simulink library "Tetris_Lib"  (R2023a)
settings: Solver=ode45  StartTime=0.0  StopTime=10.0  RelTol=1e-3  EnableMultiTasking=on
libraries: simulink_extras x33, $bdroot x16, Bit_Multiplexers_Lib x9, Decoders_Lib x4
(part 1 of 2)
settings Model: Creator=Jozko Mrkvicka  LastModifiedBy=Jozko Mrkvicka
settings SolverCC: AlgebraicLoopSolver=TrustRegion
settings DataIOCC: LimitDataPoints=on  ReturnWorkspaceOutputs=off
settings OptimizationCC: LifeSpan=inf
settings DebuggingCC: UnconnectedInputMsg=warning  UnconnectedOutputMsg=warning  UnconnectedLineMsg=warning  AllowSymbolicDim=off  SFUnexpectedBacktrackingDiag=warning  SFNoUnconditionalDefaultTransitionDiag=warning  ArithmeticOperatorsInVariantConditions=warning
settings ModelReferenceCC: EnableRefExpFcnMdlSchedulingChecks=on
settings SFSimCC: SimUseLocalCustomCode=off  CustomCodeUndefinedFunction=UseInterfaceOnly
settings RTWCC: RTWUseLocalCustomCode=off
settings CodeAppCC: StateflowObjectComments=on
settings GRTTargetCC: TargetLangStandard=C89/C90 (ANSI)
settings ConfigComp: CovMetricSettings=dw  CovSaveCumulativeToWorkspaceVar=on  CovSaveSingleToWorkspaceVar=on  CovExternalEMLEnable=off

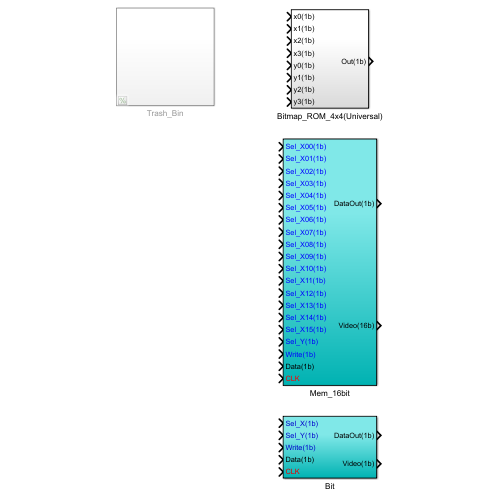
[thumbnail: Simulink's stored preview of the top-level diagram]
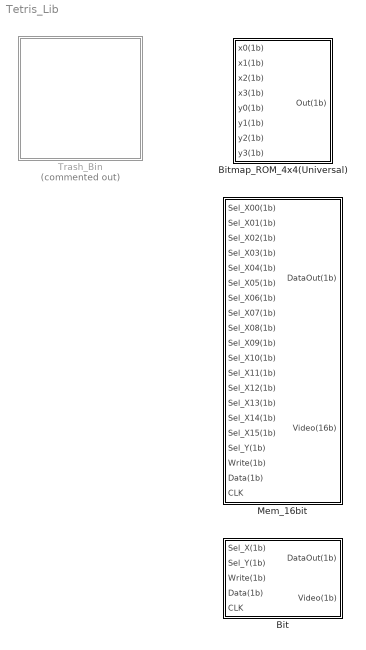
== system Tetris_Lib ==
  Bit : Subsystem
  Bitmap_ROM_4x4(Universal) : Subsystem
  Mem_16bit : Subsystem
  Trash_Bin : Subsystem  Commented=on

== system Tetris_Lib/Bit ==
  Sel_X(1b) : Inport  OutDataTypeStr=boolean
  Sel_Y(1b) : Inport  Port=2  OutDataTypeStr=boolean
  Write(1b) : Inport  Port=3  OutDataTypeStr=boolean
  Data(1b) : Inport  Port=4  OutDataTypeStr=boolean
  CLK : Inport  Port=5  OutDataTypeStr=double
  J-K Flip-Flop : simulink_extras/Flip Flops/J-K Flip-Flop  initial_condition=0
  Logical Operator : Logic  Operator=NOT  IconShape=distinctive  AllPortsSameDT=off  OutDataTypeStr=boolean
  Logical Operator1 : Logic  Inputs=3  IconShape=distinctive  AllPortsSameDT=off  OutDataTypeStr=boolean
  Logical Operator2 : Logic  Inputs=3  IconShape=distinctive  AllPortsSameDT=off  OutDataTypeStr=boolean
  Logical Operator3 : Logic  IconShape=distinctive  AllPortsSameDT=off  OutDataTypeStr=boolean
  Logical Operator4 : Logic  IconShape=distinctive  AllPortsSameDT=off  OutDataTypeStr=boolean
  Terminator : Terminator
  DataOut(1b) : Outport
  Video(1b) : Outport  Port=2
  wires:
  Write(1b)/1 -> Logical Operator1/2, Logical Operator2/2
  Logical Operator3/1 -> Logical Operator1/1, Logical Operator2/1, Logical Operator4/1
  Logical Operator4/1 -> DataOut(1b)/1
  Data(1b)/1 -> Logical Operator/1, Logical Operator1/3
  J-K Flip-Flop/2 -> Terminator/1
  J-K Flip-Flop/1 -> Logical Operator4/2, Video(1b)/1
  CLK/1 -> J-K Flip-Flop/2
  Logical Operator/1 -> Logical Operator2/3
  Logical Operator1/1 -> J-K Flip-Flop/1
  Logical Operator2/1 -> J-K Flip-Flop/3
  Sel_Y(1b)/1 -> Logical Operator3/2
  Sel_X(1b)/1 -> Logical Operator3/1

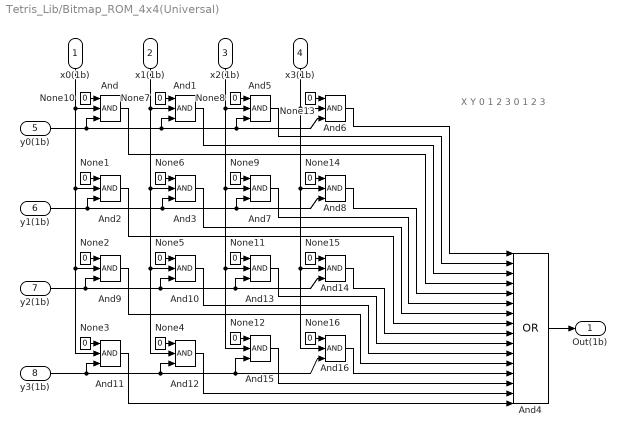
== system Tetris_Lib/Bitmap_ROM_4x4(Universal) ==
  note: X
      |
      | Y
      |
      | 0
      | 1
      | 2
      | 3
      |
      | 0
      |
      | 1
      |
      | 2
      |
      | 3
  x0(1b) : Inport
  x1(1b) : Inport  Port=2
  x2(1b) : Inport  Port=3
  x3(1b) : Inport  Port=4
  y0(1b) : Inport  Port=5
  y1(1b) : Inport  Port=6
  y2(1b) : Inport  Port=7
  y3(1b) : Inport  Port=8
  And{,1..3,5..16} (16 alike) : Logic  Inputs=3  IconShape=distinctive  AllPortsSameDT=off  OutDataTypeStr=boolean
  And4 : Logic  Operator=OR  Inputs=16  IconShape=distinctive  AllPortsSameDT=off  OutDataTypeStr=boolean
  None{1..16} (16 alike) : Constant  Value=0  OutDataTypeStr=boolean
  Out(1b) : Outport
  wires:
  y0(1b)/1 -> And/3, And1/3, And6/3, And5/3
  y1(1b)/1 -> And2/3, And3/3, And8/3, And7/3
  x0(1b)/1 -> And/2, And2/2, And11/2, And9/2
  x1(1b)/1 -> And1/2, And3/2, And12/2, And10/2
  And4/1 -> Out(1b)/1
  x2(1b)/1 -> And5/2, And7/2, And15/2, And13/2
  x3(1b)/1 -> And6/2, And8/2, And16/2, And14/2
  y2(1b)/1 -> And9/3, And10/3, And14/3, And13/3
  y3(1b)/1 -> And11/3, And12/3, And16/3, And15/3
  And6/1 -> And4/1
  And5/1 -> And4/2
  And1/1 -> And4/3
  And/1 -> And4/4
  And8/1 -> And4/5
  And7/1 -> And4/6
  And3/1 -> And4/7
  And2/1 -> And4/8
  And14/1 -> And4/9
  And13/1 -> And4/10
  And10/1 -> And4/11
  And9/1 -> And4/12
  And16/1 -> And4/13
  And15/1 -> And4/14
  And12/1 -> And4/15
  And11/1 -> And4/16
  None10/1 -> And/1
  None1/1 -> And2/1
  None2/1 -> And9/1
  None3/1 -> And11/1
  None4/1 -> And12/1
  None5/1 -> And10/1
  None6/1 -> And3/1
  None7/1 -> And1/1
  None8/1 -> And5/1
  None9/1 -> And7/1
  None11/1 -> And13/1
  None12/1 -> And15/1
  None13/1 -> And6/1
  None14/1 -> And8/1
  None15/1 -> And14/1
  None16/1 -> And16/1

== system Tetris_Lib/Mem_16bit ==
  Sel_X00(1b) : Inport
  Sel_X01(1b) : Inport  Port=2
  Sel_X02(1b) : Inport  Port=3
  Sel_X03(1b) : Inport  Port=4
  Sel_X04(1b) : Inport  Port=5
  Sel_X05(1b) : Inport  Port=6
  Sel_X06(1b) : Inport  Port=7
  Sel_X07(1b) : Inport  Port=8
  Sel_X08(1b) : Inport  Port=9
  Sel_X09(1b) : Inport  Port=10
  Sel_X10(1b) : Inport  Port=11
  Sel_X11(1b) : Inport  Port=12
  Sel_X12(1b) : Inport  Port=13
  Sel_X13(1b) : Inport  Port=14
  Sel_X14(1b) : Inport  Port=15
  Sel_X15(1b) : Inport  Port=16
  Sel_Y(1b) : Inport  Port=17
  Write(1b) : Inport  Port=18
  Data(1b) : Inport  Port=19
  CLK : Inport  Port=20
  Bit{,1..15} (16 alike) : $bdroot/Bit  SystemSampleTime=-1  VariantActivationTime=update diagram  Latency=0  AutoFrameSizeCalculation=off
  Bus Creator3 : BusCreator  Inputs=16
  Logical Operator61 : Logic  Operator=OR  Inputs=16  IconShape=distinctive  AllPortsSameDT=off  OutDataTypeStr=boolean
  DataOut(1b) : Outport
  Video(16b) : Outport  Port=2
  wires:
  Sel_Y(1b)/1 -> Bit/2, Bit15/2, Bit14/2, Bit13/2, Bit12/2, Bit11/2, Bit10/2, Bit9/2, Bit8/2, Bit7/2, Bit6/2, Bit5/2, Bit4/2, Bit3/2, Bit2/2, Bit1/2
  Data(1b)/1 -> Bit/4, Bit10/4, Bit11/4, Bit15/4, Bit14/4, Bit13/4, Bit12/4, Bit9/4, Bit8/4, Bit7/4, Bit6/4, Bit5/4, Bit4/4, Bit3/4, Bit2/4, Bit1/4
  CLK/1 -> Bit/5, Bit15/5, Bit14/5, Bit13/5, Bit12/5, Bit11/5, Bit10/5, Bit9/5, Bit8/5, Bit7/5, Bit6/5, Bit5/5, Bit4/5, Bit3/5, Bit2/5, Bit1/5
  Sel_X00(1b)/1 -> Bit/1
  Sel_X01(1b)/1 -> Bit1/1
  Sel_X02(1b)/1 -> Bit2/1
  Sel_X03(1b)/1 -> Bit3/1
  Sel_X04(1b)/1 -> Bit4/1
  Sel_X05(1b)/1 -> Bit5/1
  Sel_X06(1b)/1 -> Bit6/1
  Sel_X07(1b)/1 -> Bit7/1
  Sel_X08(1b)/1 -> Bit8/1
  Sel_X09(1b)/1 -> Bit9/1
  Sel_X10(1b)/1 -> Bit10/1
  Sel_X11(1b)/1 -> Bit11/1
  Sel_X12(1b)/1 -> Bit12/1
  Sel_X13(1b)/1 -> Bit13/1
  Sel_X14(1b)/1 -> Bit14/1
  Sel_X15(1b)/1 -> Bit15/1
  Write(1b)/1 -> Bit/3, Bit15/3, Bit14/3, Bit13/3, Bit12/3, Bit11/3, Bit10/3, Bit9/3, Bit8/3, Bit7/3, Bit6/3, Bit5/3, Bit4/3, Bit3/3, Bit2/3, Bit1/3
  Bit15/1 -> Logical Operator61/1
  Bit14/1 -> Logical Operator61/2
  Bit13/1 -> Logical Operator61/3
  Bit12/1 -> Logical Operator61/4
  Bit11/1 -> Logical Operator61/5
  Bit10/1 -> Logical Operator61/6
  Bit9/1 -> Logical Operator61/7
  Bit8/1 -> Logical Operator61/8
  Bit7/1 -> Logical Operator61/9
  Bit6/1 -> Logical Operator61/10
  Bit5/1 -> Logical Operator61/11
  Bit4/1 -> Logical Operator61/12
  Bit3/1 -> Logical Operator61/13
  Bit2/1 -> Logical Operator61/15
  Bit1/1 -> Logical Operator61/14
  Bit/1 -> Logical Operator61/16
  Bit15/2 -> Bus Creator3/16
  Bit14/2 -> Bus Creator3/15
  Bit13/2 -> Bus Creator3/14
  Bit12/2 -> Bus Creator3/13
  Bit11/2 -> Bus Creator3/12
  Bit10/2 -> Bus Creator3/11
  Bit9/2 -> Bus Creator3/10
  Bit8/2 -> Bus Creator3/9
  Bit7/2 -> Bus Creator3/8
  Bit6/2 -> Bus Creator3/7
  Bit5/2 -> Bus Creator3/6
  Bit4/2 -> Bus Creator3/5
  Bit3/2 -> Bus Creator3/4
  Bit2/2 -> Bus Creator3/3
  Bit1/2 -> Bus Creator3/2
  Bit/2 -> Bus Creator3/1
  Logical Operator61/1 -> DataOut(1b)/1
  Bus Creator3/1 -> Video(16b)/1

== system Tetris_Lib/Trash_Bin ==
  L1-Shape : Subsystem  Commented=on
  L2-Shape : Subsystem  Commented=on
  NOT_USED_I-Shape : Subsystem  Commented=on
  NOT_USED_O-Shape : Subsystem  Commented=on
  Shape_Bitmaps : Subsystem
  Subsystem1 : Subsystem
  T-Shape : Subsystem  Commented=on
  Z1-Shape : Subsystem  Commented=on
  Z2-Shape : Subsystem  Commented=on

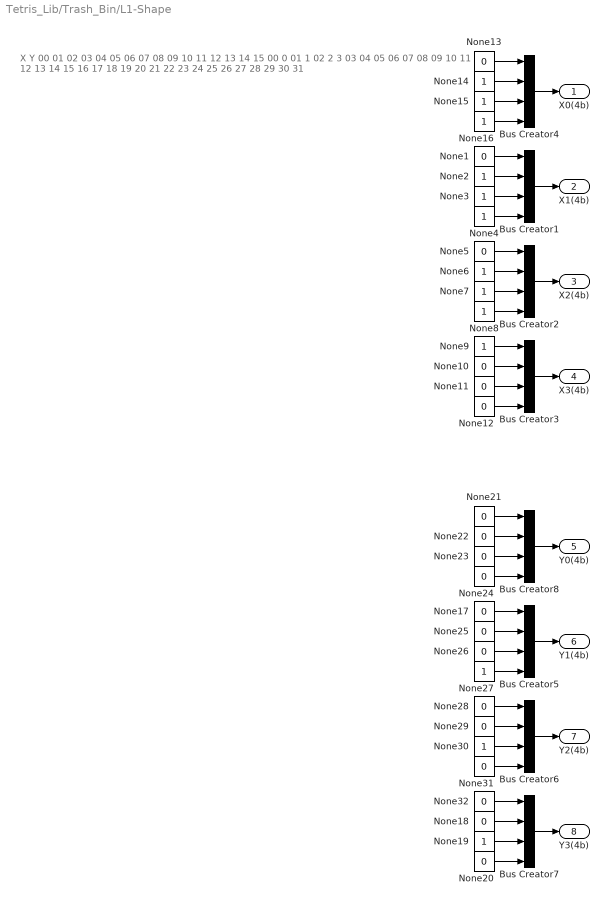
== system Tetris_Lib/Trash_Bin/L1-Shape ==
  note: X
      |
      | Y
      |
      | 00
      | 01
      | 02
      | 03
      | 04
      | 05
      | 06
      | 07
      | 08
      | 09
      | 10
      | 11
      | 12
      | 13
      | 14
      | 15
      |
      | 00
      |
      | 0
      |
      | 01
      |
      | 1
      |
      | 02
      |
      | 2
      | 3
      |
      | 03
      |
      | 04
      |
      | 05
      |
      | 06
      |
      | 07
      |
      | 08
      |
      | 09
      |
      | 10
      |
      | 11
      |
      | 12
      |
      | 13
      |
      | 14
      |
      | 15
      |
      | 16
      |
      | 17
      |
      | 18
      |
      | 19
      |
      | 20
      |
      | 21
      |
      | 22
      |
      | 23
      |
      | 24
      |
      | 25
      |
      | 26
      |
      | 27
      |
      | 28
      |
      | 29
      |
      | 30
      |
      | 31
  Bus Creator{1..8} (8 alike) : BusCreator  Inputs=4
  None{1,5,10..13,17..18,20..26,28..29,31..32} (19 alike) : Constant  Value=0  OutDataTypeStr=boolean
  None{2..4,6..9,14..16,19,27,30} (13 alike) : Constant  OutDataTypeStr=boolean
  X0(4b) : Outport
  X1(4b) : Outport  Port=2
  X2(4b) : Outport  Port=3
  X3(4b) : Outport  Port=4
  Y0(4b) : Outport  Port=5
  Y1(4b) : Outport  Port=6
  Y2(4b) : Outport  Port=7
  Y3(4b) : Outport  Port=8
  wires:
  None24/1 -> Bus Creator8/4
  None23/1 -> Bus Creator8/3
  None22/1 -> Bus Creator8/2
  None21/1 -> Bus Creator8/1
  Bus Creator8/1 -> Y0(4b)/1
  None20/1 -> Bus Creator7/4
  None19/1 -> Bus Creator7/3
  None18/1 -> Bus Creator7/2
  None32/1 -> Bus Creator7/1
  Bus Creator7/1 -> Y3(4b)/1
  None31/1 -> Bus Creator6/4
  None30/1 -> Bus Creator6/3
  None29/1 -> Bus Creator6/2
  None28/1 -> Bus Creator6/1
  Bus Creator6/1 -> Y2(4b)/1
  None27/1 -> Bus Creator5/4
  None26/1 -> Bus Creator5/3
  None25/1 -> Bus Creator5/2
  None17/1 -> Bus Creator5/1
  Bus Creator5/1 -> Y1(4b)/1
  None16/1 -> Bus Creator4/4
  None15/1 -> Bus Creator4/3
  None14/1 -> Bus Creator4/2
  None13/1 -> Bus Creator4/1
  Bus Creator4/1 -> X0(4b)/1
  None12/1 -> Bus Creator3/4
  None11/1 -> Bus Creator3/3
  None10/1 -> Bus Creator3/2
  None9/1 -> Bus Creator3/1
  Bus Creator3/1 -> X3(4b)/1
  None8/1 -> Bus Creator2/4
  None7/1 -> Bus Creator2/3
  None6/1 -> Bus Creator2/2
  None5/1 -> Bus Creator2/1
  Bus Creator2/1 -> X2(4b)/1
  None4/1 -> Bus Creator1/4
  None3/1 -> Bus Creator1/3
  None2/1 -> Bus Creator1/2
  None1/1 -> Bus Creator1/1
  Bus Creator1/1 -> X1(4b)/1

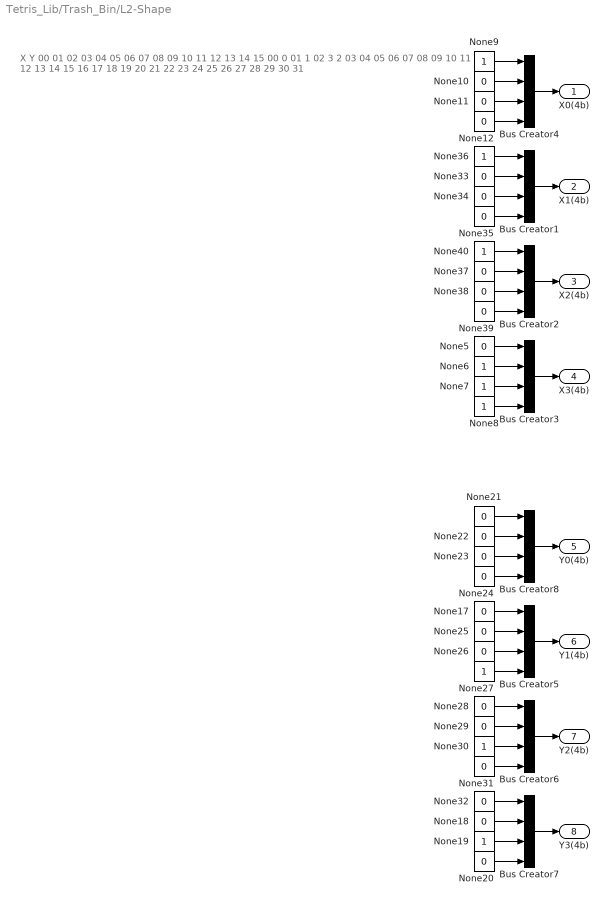
== system Tetris_Lib/Trash_Bin/L2-Shape ==
  note: X
      |
      | Y
      |
      | 00
      | 01
      | 02
      | 03
      | 04
      | 05
      | 06
      | 07
      | 08
      | 09
      | 10
      | 11
      | 12
      | 13
      | 14
      | 15
      |
      | 00
      |
      | 0
      |
      | 01
      |
      | 1
      |
      | 02
      |
      | 3
      | 2
      |
      | 03
      |
      | 04
      |
      | 05
      |
      | 06
      |
      | 07
      |
      | 08
      |
      | 09
      |
      | 10
      |
      | 11
      |
      | 12
      |
      | 13
      |
      | 14
      |
      | 15
      |
      | 16
      |
      | 17
      |
      | 18
      |
      | 19
      |
      | 20
      |
      | 21
      |
      | 22
      |
      | 23
      |
      | 24
      |
      | 25
      |
      | 26
      |
      | 27
      |
      | 28
      |
      | 29
      |
      | 30
      |
      | 31
  Bus Creator{1..8} (8 alike) : BusCreator  Inputs=4
  None{5,10..12,17..18,20..26,28..29,31..35,37..39} (23 alike) : Constant  Value=0  OutDataTypeStr=boolean
  None{6..9,19,27,30,36,40} (9 alike) : Constant  OutDataTypeStr=boolean
  X0(4b) : Outport
  X1(4b) : Outport  Port=2
  X2(4b) : Outport  Port=3
  X3(4b) : Outport  Port=4
  Y0(4b) : Outport  Port=5
  Y1(4b) : Outport  Port=6
  Y2(4b) : Outport  Port=7
  Y3(4b) : Outport  Port=8
  wires:
  None24/1 -> Bus Creator8/4
  None23/1 -> Bus Creator8/3
  None22/1 -> Bus Creator8/2
  None21/1 -> Bus Creator8/1
  Bus Creator8/1 -> Y0(4b)/1
  None20/1 -> Bus Creator7/4
  None19/1 -> Bus Creator7/3
  None18/1 -> Bus Creator7/2
  None32/1 -> Bus Creator7/1
  Bus Creator7/1 -> Y3(4b)/1
  None31/1 -> Bus Creator6/4
  None30/1 -> Bus Creator6/3
  None29/1 -> Bus Creator6/2
  None28/1 -> Bus Creator6/1
  Bus Creator6/1 -> Y2(4b)/1
  None27/1 -> Bus Creator5/4
  None26/1 -> Bus Creator5/3
  None25/1 -> Bus Creator5/2
  None17/1 -> Bus Creator5/1
  Bus Creator5/1 -> Y1(4b)/1
  None12/1 -> Bus Creator4/4
  None11/1 -> Bus Creator4/3
  None10/1 -> Bus Creator4/2
  None9/1 -> Bus Creator4/1
  Bus Creator4/1 -> X0(4b)/1
  None8/1 -> Bus Creator3/4
  None7/1 -> Bus Creator3/3
  None6/1 -> Bus Creator3/2
  None5/1 -> Bus Creator3/1
  Bus Creator3/1 -> X3(4b)/1
  None39/1 -> Bus Creator2/4
  None38/1 -> Bus Creator2/3
  None37/1 -> Bus Creator2/2
  None40/1 -> Bus Creator2/1
  Bus Creator2/1 -> X2(4b)/1
  None35/1 -> Bus Creator1/4
  None34/1 -> Bus Creator1/3
  None33/1 -> Bus Creator1/2
  None36/1 -> Bus Creator1/1
  Bus Creator1/1 -> X1(4b)/1

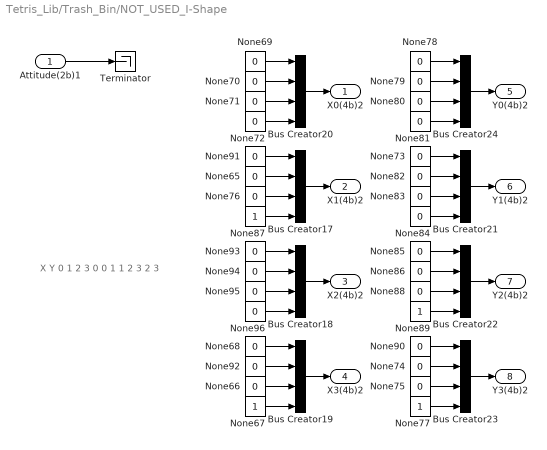
== system Tetris_Lib/Trash_Bin/NOT_USED_I-Shape ==
  note: X
      |
      | Y
      |
      | 0
      | 1
      | 2
      | 3
      |
      | 0
      | 0
      | 1
      |
      | 1
      | 2
      | 3
      |
      | 2
      |
      | 3
  Attitude(2b)1 : Inport
  Bus Creator{17..24} (8 alike) : BusCreator  Inputs=4
  None{65..66,68..76,78..86,88,90..96} (28 alike) : Constant  Value=0  OutDataTypeStr=boolean
  None{67,77,87,89} (4 alike) : Constant  OutDataTypeStr=boolean
  Terminator : Terminator
  X0(4b)2 : Outport
  X1(4b)2 : Outport  Port=2
  X2(4b)2 : Outport  Port=3
  X3(4b)2 : Outport  Port=4
  Y0(4b)2 : Outport  Port=5
  Y1(4b)2 : Outport  Port=6
  Y2(4b)2 : Outport  Port=7
  Y3(4b)2 : Outport  Port=8
  wires:
  Attitude(2b)1/1 -> Terminator/1
  None81/1 -> Bus Creator24/4
  None80/1 -> Bus Creator24/3
  None79/1 -> Bus Creator24/2
  None78/1 -> Bus Creator24/1
  Bus Creator24/1 -> Y0(4b)2/1
  None77/1 -> Bus Creator23/4
  None75/1 -> Bus Creator23/3
  None74/1 -> Bus Creator23/2
  None90/1 -> Bus Creator23/1
  Bus Creator23/1 -> Y3(4b)2/1
  None89/1 -> Bus Creator22/4
  None88/1 -> Bus Creator22/3
  None86/1 -> Bus Creator22/2
  None85/1 -> Bus Creator22/1
  Bus Creator22/1 -> Y2(4b)2/1
  None84/1 -> Bus Creator21/4
  None83/1 -> Bus Creator21/3
  None82/1 -> Bus Creator21/2
  None73/1 -> Bus Creator21/1
  Bus Creator21/1 -> Y1(4b)2/1
  None72/1 -> Bus Creator20/4
  None71/1 -> Bus Creator20/3
  None70/1 -> Bus Creator20/2
  None69/1 -> Bus Creator20/1
  Bus Creator20/1 -> X0(4b)2/1
  None67/1 -> Bus Creator19/4
  None66/1 -> Bus Creator19/3
  None92/1 -> Bus Creator19/2
  None68/1 -> Bus Creator19/1
  Bus Creator19/1 -> X3(4b)2/1
  None96/1 -> Bus Creator18/4
  None95/1 -> Bus Creator18/3
  None94/1 -> Bus Creator18/2
  None93/1 -> Bus Creator18/1
  Bus Creator18/1 -> X2(4b)2/1
  None87/1 -> Bus Creator17/4
  None76/1 -> Bus Creator17/3
  None65/1 -> Bus Creator17/2
  None91/1 -> Bus Creator17/1
  Bus Creator17/1 -> X1(4b)2/1

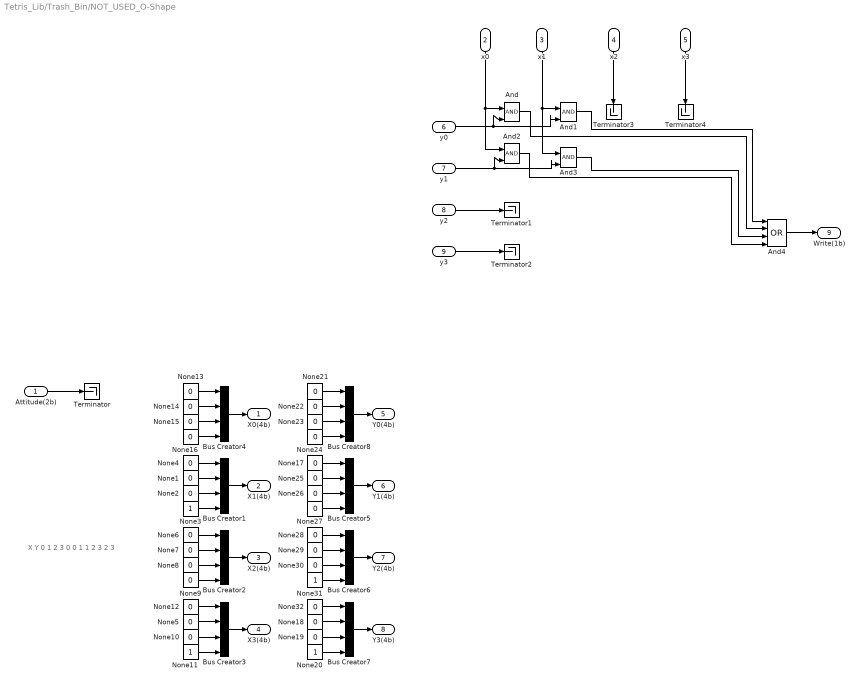
== system Tetris_Lib/Trash_Bin/NOT_USED_O-Shape ==
  note: X
      |
      | Y
      |
      | 0
      | 1
      | 2
      | 3
      |
      | 0
      | 0
      | 1
      |
      | 1
      | 2
      | 3
      |
      | 2
      |
      | 3
  Attitude(2b) : Inport
  x0 : Inport  Port=2
  x1 : Inport  Port=3
  x2 : Inport  Port=4
  x3 : Inport  Port=5
  y0 : Inport  Port=6
  y1 : Inport  Port=7
  y2 : Inport  Port=8
  y3 : Inport  Port=9
  And{,1..3} (4 alike) : Logic  IconShape=distinctive  AllPortsSameDT=off  OutDataTypeStr=boolean
  And4 : Logic  Operator=OR  Inputs=4  IconShape=distinctive  AllPortsSameDT=off  OutDataTypeStr=boolean
  Bus Creator{1..8} (8 alike) : BusCreator  Inputs=4
  None{1..2,4..10,12..19,21..30,32} (28 alike) : Constant  Value=0  OutDataTypeStr=boolean
  None{3,11,20,31} (4 alike) : Constant  OutDataTypeStr=boolean
  Terminator{,1..4} (5 alike) : Terminator
  X0(4b) : Outport
  X1(4b) : Outport  Port=2
  X2(4b) : Outport  Port=3
  X3(4b) : Outport  Port=4
  Y0(4b) : Outport  Port=5
  Y1(4b) : Outport  Port=6
  Y2(4b) : Outport  Port=7
  Y3(4b) : Outport  Port=8
  Write(1b) : Outport  Port=9
  wires:
  Attitude(2b)/1 -> Terminator/1
  None24/1 -> Bus Creator8/4
  None23/1 -> Bus Creator8/3
  None22/1 -> Bus Creator8/2
  None21/1 -> Bus Creator8/1
  Bus Creator8/1 -> Y0(4b)/1
  None20/1 -> Bus Creator7/4
  None19/1 -> Bus Creator7/3
  None18/1 -> Bus Creator7/2
  None32/1 -> Bus Creator7/1
  Bus Creator7/1 -> Y3(4b)/1
  None31/1 -> Bus Creator6/4
  None30/1 -> Bus Creator6/3
  None29/1 -> Bus Creator6/2
  None28/1 -> Bus Creator6/1
  Bus Creator6/1 -> Y2(4b)/1
  None27/1 -> Bus Creator5/4
  None26/1 -> Bus Creator5/3
  None25/1 -> Bus Creator5/2
  None17/1 -> Bus Creator5/1
  Bus Creator5/1 -> Y1(4b)/1
  None16/1 -> Bus Creator4/4
  None15/1 -> Bus Creator4/3
  None14/1 -> Bus Creator4/2
  None13/1 -> Bus Creator4/1
  Bus Creator4/1 -> X0(4b)/1
  None11/1 -> Bus Creator3/4
  None10/1 -> Bus Creator3/3
  None5/1 -> Bus Creator3/2
  None12/1 -> Bus Creator3/1
  Bus Creator3/1 -> X3(4b)/1
  None9/1 -> Bus Creator2/4
  None8/1 -> Bus Creator2/3
  None7/1 -> Bus Creator2/2
  None6/1 -> Bus Creator2/1
  Bus Creator2/1 -> X2(4b)/1
  None3/1 -> Bus Creator1/4
  None2/1 -> Bus Creator1/3
  None1/1 -> Bus Creator1/2
  None4/1 -> Bus Creator1/1
  Bus Creator1/1 -> X1(4b)/1
  y0/1 -> And/2, And1/2
  y1/1 -> And2/2, And3/2
  x0/1 -> And/1, And2/1
  x1/1 -> And1/1, And3/1
  y2/1 -> Terminator1/1
  y3/1 -> Terminator2/1
  x2/1 -> Terminator3/1
  x3/1 -> Terminator4/1
  And1/1 -> And4/1
  And/1 -> And4/2
  And3/1 -> And4/3
  And2/1 -> And4/4
  And4/1 -> Write(1b)/1

== system Tetris_Lib/Trash_Bin/Shape_Bitmaps ==
  Sel_Y(2b) : Inport
  Sel_X(2b) : Inport  Port=2
  Shape(3b) : Inport  Port=3
  Angle(2b) : Inport  Port=4
  Bus Selector1 : BusSelector  OutputSignals=signal1,signal2,signal3
  Bus Selector2 : BusSelector  OutputSignals=signal1,signal2
  Bus Selector3 : BusSelector  OutputSignals=signal3,signal4
  Bus Selector4 : BusSelector  OutputSignals=signal1,signal2
  I-shape (0deg) : Subsystem
  I-shape (90deg) : Subsystem
  L1-shape (0deg) : Subsystem
  L1-shape (180deg) : Subsystem
  L1-shape (270deg) : Subsystem
  L1-shape (90deg) : Subsystem
  L2-shape (0deg) : Subsystem
  L2-shape (180deg) : Subsystem
  L2-shape (270deg) : Subsystem
  L2-shape (90deg) : Subsystem
  None14 : Constant  Value=0  OutDataTypeStr=boolean
  O-shape : Subsystem
  Select_Angle_I : Bit_Multiplexers_Lib/Bit_Multiplexers_Lib/Bit_Multiplexer_4_to_1  SystemSampleTime=-1  VariantActivationTime=update diagram  Latency=0  AutoFrameSizeCalculation=off
  Select_Angle_L1 : Bit_Multiplexers_Lib/Bit_Multiplexers_Lib/Bit_Multiplexer_4_to_1  SystemSampleTime=-1  VariantActivationTime=update diagram  Latency=0  AutoFrameSizeCalculation=off
  Select_Angle_L2 : Bit_Multiplexers_Lib/Bit_Multiplexers_Lib/Bit_Multiplexer_4_to_1  SystemSampleTime=-1  VariantActivationTime=update diagram  Latency=0  AutoFrameSizeCalculation=off
  Select_Angle_O : Bit_Multiplexers_Lib/Bit_Multiplexers_Lib/Bit_Multiplexer_4_to_1  SystemSampleTime=-1  VariantActivationTime=update diagram  Latency=0  AutoFrameSizeCalculation=off
  Select_Angle_T : Bit_Multiplexers_Lib/Bit_Multiplexers_Lib/Bit_Multiplexer_4_to_1  SystemSampleTime=-1  VariantActivationTime=update diagram  Latency=0  AutoFrameSizeCalculation=off
  Select_Angle_Z1 : Bit_Multiplexers_Lib/Bit_Multiplexers_Lib/Bit_Multiplexer_4_to_1  SystemSampleTime=-1  VariantActivationTime=update diagram  Latency=0  AutoFrameSizeCalculation=off
  Select_Angle_Z2 : Bit_Multiplexers_Lib/Bit_Multiplexers_Lib/Bit_Multiplexer_4_to_1  SystemSampleTime=-1  VariantActivationTime=update diagram  Latency=0  AutoFrameSizeCalculation=off
  Select_Shape : Bit_Multiplexers_Lib/Bit_Multiplexers_Lib/Bit_Multiplexer_8_to_1  SystemSampleTime=-1  VariantActivationTime=update diagram  Latency=0  AutoFrameSizeCalculation=off
  Select_X : Decoders_Lib/Decoders_Lib/Decoder_2_to_4  SystemSampleTime=-1  VariantActivationTime=update diagram  Latency=0  AutoFrameSizeCalculation=off
  Select_Y : Decoders_Lib/Decoders_Lib/Decoder_2_to_4  SystemSampleTime=-1  VariantActivationTime=update diagram  Latency=0  AutoFrameSizeCalculation=off
  T-shape (0deg) : Subsystem
  T-shape (180deg) : Subsystem
  T-shape (270deg) : Subsystem
  T-shape (90deg) : Subsystem
  Z1-shape (0deg) : Subsystem
  Z1-shape (90deg) : Subsystem
  Z2-shape (0deg) : Subsystem
  Z2-shape (90deg) : Subsystem
  Pixel(1b) : Outport
  wires:
  Select_Angle_Z2/1 -> Select_Shape/8
  Select_Angle_Z1/1 -> Select_Shape/7
  I-shape (0deg)/1(Out(1b)) -> Select_Angle_I/6, Select_Angle_I/4
  Z2-shape (90deg)/1(Out(1b)) -> Select_Angle_Z2/3, Select_Angle_Z2/5
  L1-shape (0deg)/1(Out(1b)) -> Select_Angle_L1/6
  T-shape (270deg)/1(Out(1b)) -> Select_Angle_T/3
  T-shape (0deg)/1(Out(1b)) -> Select_Angle_T/6
  Z1-shape (0deg)/1(Out(1b)) -> Select_Angle_Z1/6, Select_Angle_Z1/4
  T-shape (180deg)/1(Out(1b)) -> Select_Angle_T/4
  Z1-shape (90deg)/1(Out(1b)) -> Select_Angle_Z1/5, Select_Angle_Z1/3
  L1-shape (90deg)/1(Out(1b)) -> Select_Angle_L1/5
  L1-shape (180deg)/1(Out(1b)) -> Select_Angle_L1/4
  L1-shape (270deg)/1(Out(1b)) -> Select_Angle_L1/3
  None14/1 -> Select_Shape/4
  Bus Selector2/1 -> Select_Angle_O/1, Select_Angle_Z2/1, Select_Angle_T/1, Select_Angle_L1/1, Select_Angle_L2/1, Select_Angle_Z1/1, Select_Angle_I/1  "<signal1>"
  Angle(2b)/1 -> Bus Selector2/1
  Bus Selector2/2 -> Select_Angle_O/2, Select_Angle_Z1/2, Select_Angle_Z2/2, Select_Angle_T/2, Select_Angle_L1/2, Select_Angle_L2/2, Select_Angle_I/2  "<signal2>"
  Select_Y/3 -> I-shape (0deg)/7(y1(1b)), Z1-shape (0deg)/7(y1(1b)), Z2-shape (0deg)/7(y1(1b)), T-shape (0deg)/7(y1(1b)), L1-shape (0deg)/7(y1(1b)), L2-shape (0deg)/7(y1(1b)), O-shape/7(y1(1b)), L1-shape (270deg)/7(y1(1b)), L2-shape (270deg)/7(y1(1b)), T-shape (270deg)/7(y1(1b)), L1-shape (180deg)/7(y1(1b)), L2-shape (180deg)/7(y1(1b)), T-shape (180deg)/7(y1(1b)), Z1-shape (90deg)/7(y1(1b)), Z2-shape (90deg)/7(y1(1b)), T-shape (90deg)/7(y1(1b)), L1-shape (90deg)/7(y1(1b)), L2-shape (90deg)/7(y1(1b)), I-shape (90deg)/7(y1(1b))
  Select_X/1 -> L1-shape (270deg)/1(x3(1b)), L2-shape (270deg)/1(x3(1b)), T-shape (270deg)/1(x3(1b)), L2-shape (180deg)/1(x3(1b)), L1-shape (180deg)/1(x3(1b)), T-shape (180deg)/1(x3(1b)), Z2-shape (90deg)/1(x3(1b)), T-shape (90deg)/1(x3(1b)), L1-shape (90deg)/1(x3(1b)), L2-shape (90deg)/1(x3(1b)), Z1-shape (90deg)/1(x3(1b)), I-shape (90deg)/1(x3(1b)), I-shape (0deg)/1(x3(1b)), Z1-shape (0deg)/1(x3(1b)), Z2-shape (0deg)/1(x3(1b)), T-shape (0deg)/1(x3(1b)), L1-shape (0deg)/1(x3(1b)), L2-shape (0deg)/1(x3(1b)), O-shape/1(x3(1b))
  T-shape (90deg)/1(Out(1b)) -> Select_Angle_T/5
  I-shape (90deg)/1(Out(1b)) -> Select_Angle_I/5, Select_Angle_I/3
  Sel_X(2b)/1 -> Bus Selector3/1
  Bus Selector4/1 -> Select_Y/1  "<signal1>"
  Bus Selector4/2 -> Select_Y/2  "<signal2>"
  Bus Selector3/2 -> Select_X/2  "<signal4>"
  Bus Selector1/2 -> Select_Shape/2  "<signal2>"
  Bus Selector1/1 -> Select_Shape/1  "<signal1>"
  Bus Selector1/3 -> Select_Shape/3  "<signal3>"
  Shape(3b)/1 -> Bus Selector1/1
  Select_X/3 -> L1-shape (270deg)/3(x1(1b)), L2-shape (270deg)/3(x1(1b)), T-shape (270deg)/3(x1(1b)), L1-shape (180deg)/3(x1(1b)), L2-shape (180deg)/3(x1(1b)), T-shape (180deg)/3(x1(1b)), Z1-shape (90deg)/3(x1(1b)), Z2-shape (90deg)/3(x1(1b)), T-shape (90deg)/3(x1(1b)), L1-shape (90deg)/3(x1(1b)), L2-shape (90deg)/3(x1(1b)), I-shape (90deg)/3(x1(1b)), I-shape (0deg)/3(x1(1b)), Z1-shape (0deg)/3(x1(1b)), Z2-shape (0deg)/3(x1(1b)), T-shape (0deg)/3(x1(1b)), L1-shape (0deg)/3(x1(1b)), L2-shape (0deg)/3(x1(1b)), O-shape/3(x1(1b))
  Select_X/4 -> L1-shape (180deg)/4(x0(1b)), L2-shape (180deg)/4(x0(1b)), T-shape (180deg)/4(x0(1b)), L1-shape (270deg)/4(x0(1b)), L2-shape (270deg)/4(x0(1b)), T-shape (270deg)/4(x0(1b)), Z1-shape (90deg)/4(x0(1b)), Z2-shape (90deg)/4(x0(1b)), T-shape (90deg)/4(x0(1b)), L1-shape (90deg)/4(x0(1b)), L2-shape (90deg)/4(x0(1b)), I-shape (90deg)/4(x0(1b)), I-shape (0deg)/4(x0(1b)), Z1-shape (0deg)/4(x0(1b)), Z2-shape (0deg)/4(x0(1b)), T-shape (0deg)/4(x0(1b)), L1-shape (0deg)/4(x0(1b)), L2-shape (0deg)/4(x0(1b)), O-shape/4(x0(1b))
  Select_Y/4 -> L1-shape (270deg)/8(y0(1b)), L2-shape (270deg)/8(y0(1b)), T-shape (270deg)/8(y0(1b)), L1-shape (180deg)/8(y0(1b)), L2-shape (180deg)/8(y0(1b)), T-shape (180deg)/8(y0(1b)), Z1-shape (90deg)/8(y0(1b)), Z2-shape (90deg)/8(y0(1b)), T-shape (90deg)/8(y0(1b)), L1-shape (90deg)/8(y0(1b)), L2-shape (90deg)/8(y0(1b)), I-shape (90deg)/8(y0(1b)), I-shape (0deg)/8(y0(1b)), Z1-shape (0deg)/8(y0(1b)), Z2-shape (0deg)/8(y0(1b)), T-shape (0deg)/8(y0(1b)), L1-shape (0deg)/8(y0(1b)), L2-shape (0deg)/8(y0(1b)), O-shape/8(y0(1b))
  Select_Y/1 -> I-shape (0deg)/5(y3(1b)), Z1-shape (0deg)/5(y3(1b)), Z2-shape (0deg)/5(y3(1b)), T-shape (0deg)/5(y3(1b)), L1-shape (0deg)/5(y3(1b)), L2-shape (0deg)/5(y3(1b)), O-shape/5(y3(1b)), L1-shape (270deg)/5(y3(1b)), L2-shape (270deg)/5(y3(1b)), T-shape (270deg)/5(y3(1b)), L1-shape (180deg)/5(y3(1b)), L2-shape (180deg)/5(y3(1b)), T-shape (180deg)/5(y3(1b)), Z1-shape (90deg)/5(y3(1b)), Z2-shape (90deg)/5(y3(1b)), T-shape (90deg)/5(y3(1b)), L1-shape (90deg)/5(y3(1b)), L2-shape (90deg)/5(y3(1b)), I-shape (90deg)/5(y3(1b))
  O-shape/1(Out(1b)) -> Select_Angle_O/6, Select_Angle_O/5, Select_Angle_O/4, Select_Angle_O/3
  L2-shape (0deg)/1(Out(1b)) -> Select_Angle_L2/6
  L2-shape (270deg)/1(Out(1b)) -> Select_Angle_L2/3
  L2-shape (180deg)/1(Out(1b)) -> Select_Angle_L2/4
  L2-shape (90deg)/1(Out(1b)) -> Select_Angle_L2/5
  Select_Y/2 -> L1-shape (270deg)/6(y2(1b)), L2-shape (270deg)/6(y2(1b)), T-shape (270deg)/6(y2(1b)), L1-shape (180deg)/6(y2(1b)), L2-shape (180deg)/6(y2(1b)), T-shape (180deg)/6(y2(1b)), Z1-shape (90deg)/6(y2(1b)), Z2-shape (90deg)/6(y2(1b)), T-shape (90deg)/6(y2(1b)), L1-shape (90deg)/6(y2(1b)), L2-shape (90deg)/6(y2(1b)), I-shape (90deg)/6(y2(1b)), I-shape (0deg)/6(y2(1b)), Z1-shape (0deg)/6(y2(1b)), Z2-shape (0deg)/6(y2(1b)), T-shape (0deg)/6(y2(1b)), L1-shape (0deg)/6(y2(1b)), L2-shape (0deg)/6(y2(1b)), O-shape/6(y2(1b))
  Select_X/2 -> I-shape (0deg)/2(x2(1b)), Z1-shape (0deg)/2(x2(1b)), Z2-shape (0deg)/2(x2(1b)), T-shape (0deg)/2(x2(1b)), L1-shape (0deg)/2(x2(1b)), L2-shape (0deg)/2(x2(1b)), O-shape/2(x2(1b)), L1-shape (270deg)/2(x2(1b)), L2-shape (270deg)/2(x2(1b)), T-shape (270deg)/2(x2(1b)), L1-shape (180deg)/2(x2(1b)), L2-shape (180deg)/2(x2(1b)), T-shape (180deg)/2(x2(1b)), Z1-shape (90deg)/2(x2(1b)), Z2-shape (90deg)/2(x2(1b)), T-shape (90deg)/2(x2(1b)), L1-shape (90deg)/2(x2(1b)), L2-shape (90deg)/2(x2(1b)), I-shape (90deg)/2(x2(1b))
  Z2-shape (0deg)/1(Out(1b)) -> Select_Angle_Z2/6, Select_Angle_Z2/4
  Select_Angle_L1/1 -> Select_Shape/10
  Select_Angle_O/1 -> Select_Shape/5
  Select_Angle_I/1 -> Select_Shape/6
  Select_Angle_L2/1 -> Select_Shape/11
  Select_Shape/1 -> Pixel(1b)/1
  Select_Angle_T/1 -> Select_Shape/9
  Bus Selector3/1 -> Select_X/1  "<signal3>"
  Sel_Y(2b)/1 -> Bus Selector4/1

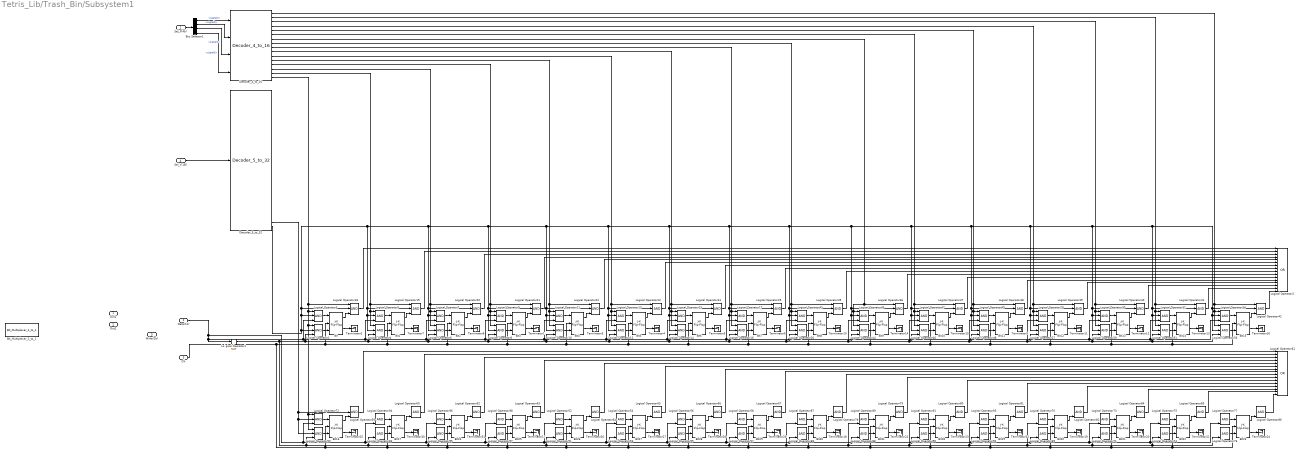
== system Tetris_Lib/Trash_Bin/Subsystem1 ==
  Sel_X(4b) : Inport
  Data(1b) : Inport  Port=2
  Clk : Inport  Port=3
  Sel_Y(1B) : Inport  Port=4
  Write(1b) : Inport  Port=5
  Bit{,1..31} (32 alike) : simulink_extras/Flip Flops/J-K Flip-Flop  initial_condition=0
  Bit_Multiplexer_2_to_1 : Bit_Multiplexers_Lib/Bit_Multiplexers_Lib/Bit_Multiplexer_2_to_1  SystemSampleTime=-1  VariantActivationTime=update diagram  Latency=0  AutoFrameSizeCalculation=off
  Bus Selector1 : BusSelector  OutputSignals=signal2,signal3,signal4,signal5
  Decoder_4_to_16 : Decoders_Lib/Decoders_Lib/Decoder_4_to_16  SystemSampleTime=-1  VariantActivationTime=update diagram  Latency=0  AutoFrameSizeCalculation=off
  Decoder_5_to_32 : Decoders_Lib/Decoders_Lib/Decoder_5_to_32  SystemSampleTime=-1  VariantActivationTime=update diagram  Latency=0  AutoFrameSizeCalculation=off
  Lo`gical Operator1 : Logic  Operator=NOT  IconShape=distinctive  AllPortsSameDT=off  OutDataTypeStr=boolean
  Logical Operator{1,3..60,62..98} (96 alike) : Logic  Inputs=3  IconShape=distinctive  AllPortsSameDT=off  OutDataTypeStr=boolean
  Logical Operator2 : Logic  Operator=OR  Inputs=16  IconShape=distinctive  AllPortsSameDT=off  OutDataTypeStr=boolean
  Logical Operator61 : Logic  Operator=OR  Inputs=16  IconShape=distinctive  AllPortsSameDT=off  OutDataTypeStr=boolean
  Terminator{1..32} (32 alike) : Terminator
  Out1 : Outport
  Out2 : Outport  Port=2
  wires:
  Bus Selector1/1 -> Decoder_4_to_16/1  "<signal2>"
  Bus Selector1/2 -> Decoder_4_to_16/2  "<signal3>"
  Bus Selector1/3 -> Decoder_4_to_16/3  "<signal4>"
  Bus Selector1/4 -> Decoder_4_to_16/4  "<signal5>"
  Sel_X(4b)/1 -> Bus Selector1/1
  Sel_Y(1B)/1 -> Decoder_5_to_32/1
  Decoder_4_to_16/16 -> Logical Operator18/1, Logical Operator72/1, Logical Operator50/1, Logical Operator1/1, Logical Operator3/1
  Logical Operator1/1 -> Bit/3
  Logical Operator3/1 -> Bit/1
  Logical Operator4/1 -> Bit1/3
  Logical Operator5/1 -> Bit1/1
  Logical Operator6/1 -> Bit2/3
  Logical Operator7/1 -> Bit2/1
  Logical Operator8/1 -> Bit3/3
  Logical Operator9/1 -> Bit3/1
  Logical Operator10/1 -> Bit4/3
  Logical Operator11/1 -> Bit4/1
  Logical Operator12/1 -> Bit5/3
  Logical Operator13/1 -> Bit5/1
  Logical Operator14/1 -> Bit6/3
  Logical Operator15/1 -> Bit6/1
  Logical Operator16/1 -> Bit7/3
  Logical Operator17/1 -> Bit7/1
  Bit/1 -> Logical Operator18/3
  Bit/2 -> Terminator2/1
  Decoder_4_to_16/15 -> Logical Operator19/1, Logical Operator5/1, Logical Operator4/1
  Bit1/1 -> Logical Operator19/3
  Decoder_4_to_16/14 -> Logical Operator20/1, Logical Operator7/1, Logical Operator6/1
  Bit2/1 -> Logical Operator20/3
  Decoder_4_to_16/13 -> Logical Operator21/1, Logical Operator8/1, Logical Operator9/1
  Bit3/1 -> Logical Operator21/3
  Bit3/2 -> Terminator1/1
  Decoder_4_to_16/12 -> Logical Operator22/1, Logical Operator10/1, Logical Operator11/1
  Bit4/1 -> Logical Operator22/3
  Bit4/2 -> Terminator3/1
  Decoder_4_to_16/11 -> Logical Operator23/1, Logical Operator13/1, Logical Operator12/1
  Bit5/1 -> Logical Operator23/3
  Bit5/2 -> Terminator4/1
  Decoder_4_to_16/10 -> Logical Operator24/1, Logical Operator15/1, Logical Operator14/1
  Bit6/1 -> Logical Operator24/3
  Bit6/2 -> Terminator5/1
  Decoder_4_to_16/9 -> Logical Operator25/1, Logical Operator16/1, Logical Operator17/1
  Bit7/1 -> Logical Operator25/3
  Bit7/2 -> Terminator6/1
  Bit1/2 -> Terminator7/1
  Bit2/2 -> Terminator8/1
  Logical Operator25/1 -> Logical Operator2/8
  Logical Operator24/1 -> Logical Operator2/7
  Logical Operator23/1 -> Logical Operator2/6
  Logical Operator22/1 -> Logical Operator2/5
  Logical Operator21/1 -> Logical Operator2/4
  Logical Operator20/1 -> Logical Operator2/3
  Logical Operator19/1 -> Logical Operator2/2
  Logical Operator18/1 -> Logical Operator2/1
  Decoder_4_to_16/8 -> Logical Operator35/1, Logical Operator26/1, Logical Operator43/1
  Logical Operator26/1 -> Bit8/3
  Logical Operator43/1 -> Bit8/1
  Logical Operator44/1 -> Bit9/3
  Logical Operator45/1 -> Bit9/1
  Logical Operator46/1 -> Bit10/3
  Logical Operator47/1 -> Bit10/1
  Logical Operator48/1 -> Bit11/3
  Logical Operator49/1 -> Bit11/1
  Logical Operator27/1 -> Bit12/3
  Logical Operator28/1 -> Bit12/1
  Logical Operator29/1 -> Bit13/3
  Logical Operator30/1 -> Bit13/1
  Logical Operator31/1 -> Bit14/3
  Logical Operator32/1 -> Bit14/1
  Logical Operator33/1 -> Bit15/3
  Logical Operator34/1 -> Bit15/1
  Bit8/1 -> Logical Operator35/3
  Bit8/2 -> Terminator10/1
  Decoder_4_to_16/7 -> Logical Operator45/1, Logical Operator44/1, Logical Operator36/1
  Bit9/1 -> Logical Operator36/3
  Decoder_4_to_16/6 -> Logical Operator37/1, Logical Operator47/1, Logical Operator46/1
  Bit10/1 -> Logical Operator37/3
  Decoder_4_to_16/5 -> Logical Operator38/1, Logical Operator48/1, Logical Operator49/1
  Bit11/1 -> Logical Operator38/3
  Bit11/2 -> Terminator9/1
  Decoder_4_to_16/4 -> Logical Operator39/1, Logical Operator27/1, Logical Operator28/1
  Bit12/1 -> Logical Operator39/3
  Bit12/2 -> Terminator11/1
  Decoder_4_to_16/3 -> Logical Operator40/1, Logical Operator30/1, Logical Operator29/1
  Bit13/1 -> Logical Operator40/3
  Bit13/2 -> Terminator12/1
  Decoder_4_to_16/2 -> Logical Operator41/1, Logical Operator32/1, Logical Operator31/1
  Bit14/1 -> Logical Operator41/3
  Bit14/2 -> Terminator13/1
  Decoder_4_to_16/1 -> Logical Operator42/1, Logical Operator33/1, Logical Operator34/1
  Bit15/1 -> Logical Operator42/3
  Bit15/2 -> Terminator16/1
  Bit9/2 -> Terminator14/1
  Bit10/2 -> Terminator15/1
  Logical Operator41/1 -> Logical Operator2/15
  Logical Operator40/1 -> Logical Operator2/14
  Logical Operator39/1 -> Logical Operator2/13
  Logical Operator38/1 -> Logical Operator2/12
  Logical Operator37/1 -> Logical Operator2/11
  Logical Operator36/1 -> Logical Operator2/10
  Logical Operator35/1 -> Logical Operator2/9
  Logical Operator42/1 -> Logical Operator2/16
  Logical Operator50/1 -> Bit16/3
  Logical Operator72/1 -> Bit16/1
  Logical Operator83/1 -> Bit17/3
  Logical Operator94/1 -> Bit17/1
  Logical Operator95/1 -> Bit24/3
  Logical Operator96/1 -> Bit24/1
  Logical Operator97/1 -> Bit25/3
  Logical Operator98/1 -> Bit25/1
  Logical Operator51/1 -> Bit26/3
  Logical Operator52/1 -> Bit26/1
  Logical Operator53/1 -> Bit27/3
  Logical Operator54/1 -> Bit27/1
  Logical Operator55/1 -> Bit28/3
  Logical Operator56/1 -> Bit28/1
  Logical Operator57/1 -> Bit29/3
  Logical Operator58/1 -> Bit29/1
  Bit16/1 -> Logical Operator59/3
  Bit16/2 -> Terminator25/1
  Bit17/1 -> Logical Operator60/3
  Bit24/1 -> Logical Operator62/3
  Bit25/1 -> Logical Operator63/3
  Bit25/2 -> Terminator17/1
  Bit26/1 -> Logical Operator64/3
  Bit26/2 -> Terminator26/1
  Bit27/1 -> Logical Operator65/3
  Bit27/2 -> Terminator27/1
  Bit28/1 -> Logical Operator66/3
  Bit28/2 -> Terminator28/1
  Bit29/1 -> Logical Operator67/3
  Bit29/2 -> Terminator29/1
  Bit17/2 -> Terminator30/1
  Bit24/2 -> Terminator31/1
  Logical Operator67/1 -> Logical Operator61/8
  Logical Operator66/1 -> Logical Operator61/7
  Logical Operator65/1 -> Logical Operator61/6
  Logical Operator64/1 -> Logical Operator61/5
  Logical Operator63/1 -> Logical Operator61/4
  Logical Operator62/1 -> Logical Operator61/3
  Logical Operator60/1 -> Logical Operator61/2
  Logical Operator59/1 -> Logical Operator61/1
  Logical Operator68/1 -> Bit30/3
  Logical Operator87/1 -> Bit30/1
  Logical Operator88/1 -> Bit31/3
  Logical Operator89/1 -> Bit31/1
  Logical Operator90/1 -> Bit18/3
  Logical Operator91/1 -> Bit18/1
  Logical Operator92/1 -> Bit19/3
  Logical Operator93/1 -> Bit19/1
  Logical Operator69/1 -> Bit20/3
  Logical Operator70/1 -> Bit20/1
  Logical Operator71/1 -> Bit21/3
  Logical Operator73/1 -> Bit21/1
  Logical Operator74/1 -> Bit22/3
  Logical Operator75/1 -> Bit22/1
  Logical Operator76/1 -> Bit23/3
  Logical Operator77/1 -> Bit23/1
  Bit30/1 -> Logical Operator78/3
  Bit30/2 -> Terminator18/1
  Bit31/1 -> Logical Operator79/3
  Bit18/1 -> Logical Operator80/3
  Bit19/1 -> Logical Operator81/3
  Bit19/2 -> Terminator32/1
  Bit20/1 -> Logical Operator82/3
  Bit20/2 -> Terminator19/1
  Bit21/1 -> Logical Operator84/3
  Bit21/2 -> Terminator20/1
  Bit22/1 -> Logical Operator85/3
  Bit22/2 -> Terminator21/1
  Decoder_5_to_32/32 -> Logical Operator35/2, Logical Operator43/2, Logical Operator26/2, Logical Operator36/2, Logical Operator45/2, Logical Operator44/2, Logical Operator37/2, Logical Operator47/2, Logical Operator46/2, Logical Operator49/2, Logical Operator48/2, Logical Operator38/2, Logical Operator39/2, Logical Operator28/2, Logical Operator27/2, Logical Operator40/2, Logical Operator30/2, Logical Operator29/2, Logical Operator41/2, Logical Operator32/2, Logical Operator31/2, Logical Operator42/2, Logical Operator34/2, Logical Operator33/2, Logical Operator25/2, Logical Operator17/2, Logical Operator16/2, Logical Operator24/2, Logical Operator15/2, Logical Operator14/2, Logical Operator23/2, Logical Operator13/2, Logical Operator12/2, Logical Operator22/2, Logical Operator11/2, Logical Operator10/2, Logical Operator21/2, Logical Operator9/2, Logical Operator8/2, Logical Operator20/2, Logical Operator7/2, Logical Operator6/2, Logical Operator19/2, Logical Operator5/2, Logical Operator4/2, Logical Operator18/2, Logical Operator3/2, Logical Operator1/2
  ? -> Logical Operator60/2, Logical Operator94/2, Logical Operator83/2
  ? -> Logical Operator62/2, Logical Operator96/2, Logical Operator95/2
  ? -> Logical Operator63/2, Logical Operator98/2, Logical Operator97/2
  ? -> Logical Operator64/2, Logical Operator52/2, Logical Operator51/2
  ? -> Logical Operator65/2, Logical Operator54/2, Logical Operator53/2
  ? -> Logical Operator66/2, Logical Operator56/2, Logical Operator55/2
  ? -> Logical Operator67/2, Logical Operator58/2, Logical Operator57/2
  ? -> Logical Operator78/2, Logical Operator87/2, Logical Operator68/2
  ? -> Logical Operator79/2, Logical Operator89/2, Logical Operator88/2
  ? -> Logical Operator80/2, Logical Operator91/2, Logical Operator90/2
  ? -> Logical Operator93/2, Logical Operator92/2, Logical Operator81/2
  ? -> Logical Operator82/2, Logical Operator70/2, Logical Operator69/2
  ? -> Logical Operator84/2, Logical Operator73/2, Logical Operator71/2
  ? -> Logical Operator86/2, Logical Operator77/2, Logical Operator76/2
  ? -> Logical Operator85/2, Logical Operator75/2, Logical Operator74/2
  Bit23/1 -> Logical Operator86/3
  Bit23/2 -> Terminator24/1
  Bit31/2 -> Terminator22/1
  Bit18/2 -> Terminator23/1
  Logical Operator85/1 -> Logical Operator61/15
  Logical Operator84/1 -> Logical Operator61/14
  Logical Operator82/1 -> Logical Operator61/13
  Logical Operator81/1 -> Logical Operator61/12
  Logical Operator80/1 -> Logical Operator61/11
  Logical Operator79/1 -> Logical Operator61/10
  Logical Operator78/1 -> Logical Operator61/9
  Logical Operator86/1 -> Logical Operator61/16
  Lo`gical Operator1/1 -> Logical Operator4/3, Logical Operator6/3, Logical Operator8/3, Logical Operator10/3, Logical Operator12/3, Logical Operator14/3, Logical Operator16/3, Logical Operator43/3, Logical Operator45/3, Logical Operator47/3, Logical Operator49/3, Logical Operator28/3, Logical Operator29/3, Logical Operator31/3, Logical Operator33/3, Logical Operator1/3, Logical Operator50/3, Logical Operator83/3, Logical Operator95/3, Logical Operator97/3, Logical Operator51/3, Logical Operator53/3, Logical Operator55/3, Logical Operator57/3, Logical Operator87/3, Logical Operator89/3, Logical Operator91/3, Logical Operator93/3, Logical Operator70/3, Logical Operator71/3, Logical Operator74/3, Logical Operator76/3
  Data(1b)/1 -> Lo`gical Operator1/1, Logical Operator3/3, Logical Operator5/3, Logical Operator7/3, Logical Operator9/3, Logical Operator11/3, Logical Operator13/3, Logical Operator15/3, Logical Operator17/3, Logical Operator26/3, Logical Operator44/3, Logical Operator46/3, Logical Operator48/3, Logical Operator27/3, Logical Operator30/3, Logical Operator34/3, Logical Operator32/3, Logical Operator72/3, Logical Operator94/3, Logical Operator96/3, Logical Operator98/3, Logical Operator52/3, Logical Operator54/3, Logical Operator56/3, Logical Operator58/3, Logical Operator68/3, Logical Operator88/3, Logical Operator90/3, Logical Operator92/3, Logical Operator69/3, Logical Operator73/3, Logical Operator77/3, Logical Operator75/3
  Clk/1 -> Bit16/2, Bit17/2, Bit24/2, Bit25/2, Bit26/2, Bit27/2, Bit28/2, Bit29/2, Bit30/2, Bit31/2, Bit18/2, Bit19/2, Bit20/2, Bit21/2, Bit22/2, Bit23/2, Bit/2, Bit1/2, Bit2/2, Bit3/2, Bit4/2, Bit5/2, Bit6/2, Bit7/2, Bit8/2, Bit9/2, Bit10/2, Bit11/2, Bit12/2, Bit13/2, Bit14/2, Bit15/2
  Decoder_5_to_32/31 -> Logical Operator72/2, Logical Operator50/2, Logical Operator59/2

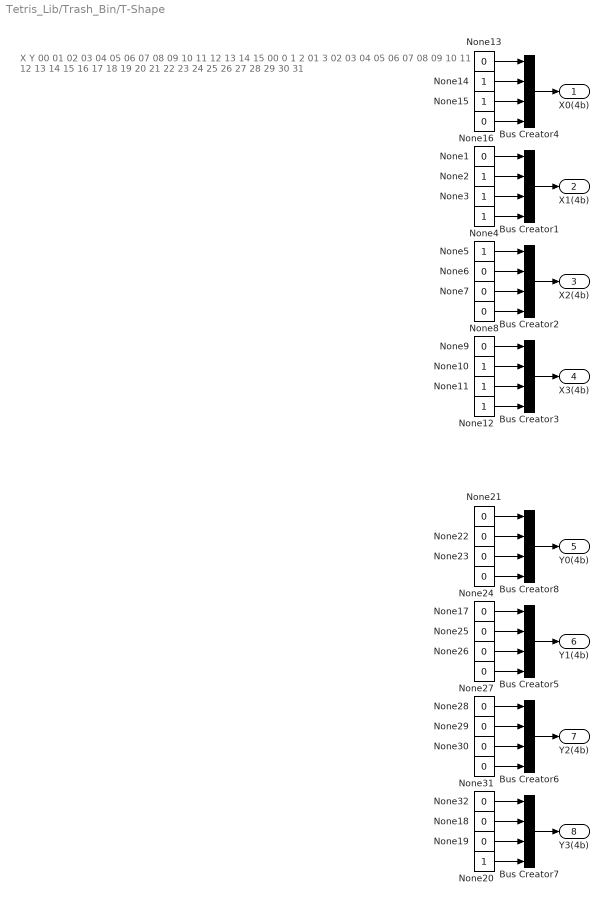
== system Tetris_Lib/Trash_Bin/T-Shape ==
  note: X
      |
      | Y
      |
      | 00
      | 01
      | 02
      | 03
      | 04
      | 05
      | 06
      | 07
      | 08
      | 09
      | 10
      | 11
      | 12
      | 13
      | 14
      | 15
      |
      | 00
      |
      | 0
      | 1
      | 2
      |
      | 01
      |
      | 3
      |
      | 02
      |
      | 03
      |
      | 04
      |
      | 05
      |
      | 06
      |
      | 07
      |
      | 08
      |
      | 09
      |
      | 10
      |
      | 11
      |
      | 12
      |
      | 13
      |
      | 14
      |
      | 15
      |
      | 16
      |
      | 17
      |
      | 18
      |
      | 19
      |
      | 20
      |
      | 21
      |
      | 22
      |
      | 23
      |
      | 24
      |
      | 25
      |
      | 26
      |
      | 27
      |
      | 28
      |
      | 29
      |
      | 30
      |
      | 31
  Bus Creator{1..8} (8 alike) : BusCreator  Inputs=4
  None{1,6..9,13,16..19,21..32} (22 alike) : Constant  Value=0  OutDataTypeStr=boolean
  None{2..5,10..12,14..15,20} (10 alike) : Constant  OutDataTypeStr=boolean
  X0(4b) : Outport
  X1(4b) : Outport  Port=2
  X2(4b) : Outport  Port=3
  X3(4b) : Outport  Port=4
  Y0(4b) : Outport  Port=5
  Y1(4b) : Outport  Port=6
  Y2(4b) : Outport  Port=7
  Y3(4b) : Outport  Port=8
  wires:
  None24/1 -> Bus Creator8/4
  None23/1 -> Bus Creator8/3
  None22/1 -> Bus Creator8/2
  None21/1 -> Bus Creator8/1
  Bus Creator8/1 -> Y0(4b)/1
  None20/1 -> Bus Creator7/4
  None19/1 -> Bus Creator7/3
  None18/1 -> Bus Creator7/2
  None32/1 -> Bus Creator7/1
  Bus Creator7/1 -> Y3(4b)/1
  None31/1 -> Bus Creator6/4
  None30/1 -> Bus Creator6/3
  None29/1 -> Bus Creator6/2
  None28/1 -> Bus Creator6/1
  Bus Creator6/1 -> Y2(4b)/1
  None27/1 -> Bus Creator5/4
  None26/1 -> Bus Creator5/3
  None25/1 -> Bus Creator5/2
  None17/1 -> Bus Creator5/1
  Bus Creator5/1 -> Y1(4b)/1
  None16/1 -> Bus Creator4/4
  None15/1 -> Bus Creator4/3
  None14/1 -> Bus Creator4/2
  None13/1 -> Bus Creator4/1
  Bus Creator4/1 -> X0(4b)/1
  None12/1 -> Bus Creator3/4
  None11/1 -> Bus Creator3/3
  None10/1 -> Bus Creator3/2
  None9/1 -> Bus Creator3/1
  Bus Creator3/1 -> X3(4b)/1
  None8/1 -> Bus Creator2/4
  None7/1 -> Bus Creator2/3
  None6/1 -> Bus Creator2/2
  None5/1 -> Bus Creator2/1
  Bus Creator2/1 -> X2(4b)/1
  None4/1 -> Bus Creator1/4
  None3/1 -> Bus Creator1/3
  None2/1 -> Bus Creator1/2
  None1/1 -> Bus Creator1/1
  Bus Creator1/1 -> X1(4b)/1

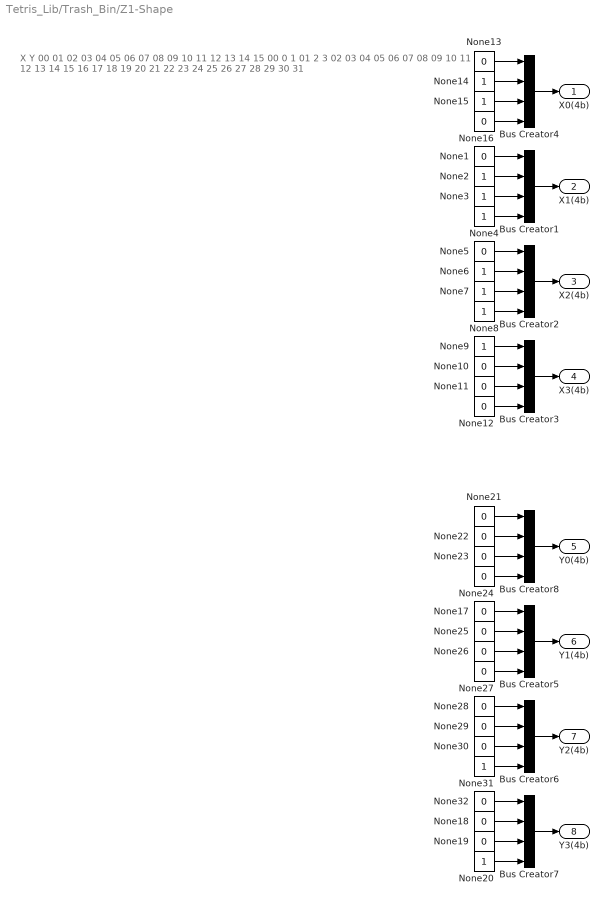
== system Tetris_Lib/Trash_Bin/Z1-Shape ==
  note: X
      |
      | Y
      |
      | 00
      | 01
      | 02
      | 03
      | 04
      | 05
      | 06
      | 07
      | 08
      | 09
      | 10
      | 11
      | 12
      | 13
      | 14
      | 15
      |
      | 00
      |
      | 0
      | 1
      |
      | 01
      |
      | 2
      | 3
      |
      | 02
      |
      | 03
      |
      | 04
      |
      | 05
      |
      | 06
      |
      | 07
      |
      | 08
      |
      | 09
      |
      | 10
      |
      | 11
      |
      | 12
      |
      | 13
      |
      | 14
      |
      | 15
      |
      | 16
      |
      | 17
      |
      | 18
      |
      | 19
      |
      | 20
      |
      | 21
      |
      | 22
      |
      | 23
      |
      | 24
      |
      | 25
      |
      | 26
      |
      | 27
      |
      | 28
      |
      | 29
      |
      | 30
      |
      | 31
  Bus Creator{1..8} (8 alike) : BusCreator  Inputs=4
  None{1,5,10..13,16..19,21..30,32} (21 alike) : Constant  Value=0  OutDataTypeStr=boolean
  None{2..4,6..9,14..15,20,31} (11 alike) : Constant  OutDataTypeStr=boolean
  X0(4b) : Outport
  X1(4b) : Outport  Port=2
  X2(4b) : Outport  Port=3
  X3(4b) : Outport  Port=4
  Y0(4b) : Outport  Port=5
  Y1(4b) : Outport  Port=6
  Y2(4b) : Outport  Port=7
  Y3(4b) : Outport  Port=8
  wires:
  None24/1 -> Bus Creator8/4
  None23/1 -> Bus Creator8/3
  None22/1 -> Bus Creator8/2
  None21/1 -> Bus Creator8/1
  Bus Creator8/1 -> Y0(4b)/1
  None20/1 -> Bus Creator7/4
  None19/1 -> Bus Creator7/3
  None18/1 -> Bus Creator7/2
  None32/1 -> Bus Creator7/1
  Bus Creator7/1 -> Y3(4b)/1
  None31/1 -> Bus Creator6/4
  None30/1 -> Bus Creator6/3
  None29/1 -> Bus Creator6/2
  None28/1 -> Bus Creator6/1
  Bus Creator6/1 -> Y2(4b)/1
  None27/1 -> Bus Creator5/4
  None26/1 -> Bus Creator5/3
  None25/1 -> Bus Creator5/2
  None17/1 -> Bus Creator5/1
  Bus Creator5/1 -> Y1(4b)/1
  None16/1 -> Bus Creator4/4
  None15/1 -> Bus Creator4/3
  None14/1 -> Bus Creator4/2
  None13/1 -> Bus Creator4/1
  Bus Creator4/1 -> X0(4b)/1
  None12/1 -> Bus Creator3/4
  None11/1 -> Bus Creator3/3
  None10/1 -> Bus Creator3/2
  None9/1 -> Bus Creator3/1
  Bus Creator3/1 -> X3(4b)/1
  None8/1 -> Bus Creator2/4
  None7/1 -> Bus Creator2/3
  None6/1 -> Bus Creator2/2
  None5/1 -> Bus Creator2/1
  Bus Creator2/1 -> X2(4b)/1
  None4/1 -> Bus Creator1/4
  None3/1 -> Bus Creator1/3
  None2/1 -> Bus Creator1/2
  None1/1 -> Bus Creator1/1
  Bus Creator1/1 -> X1(4b)/1

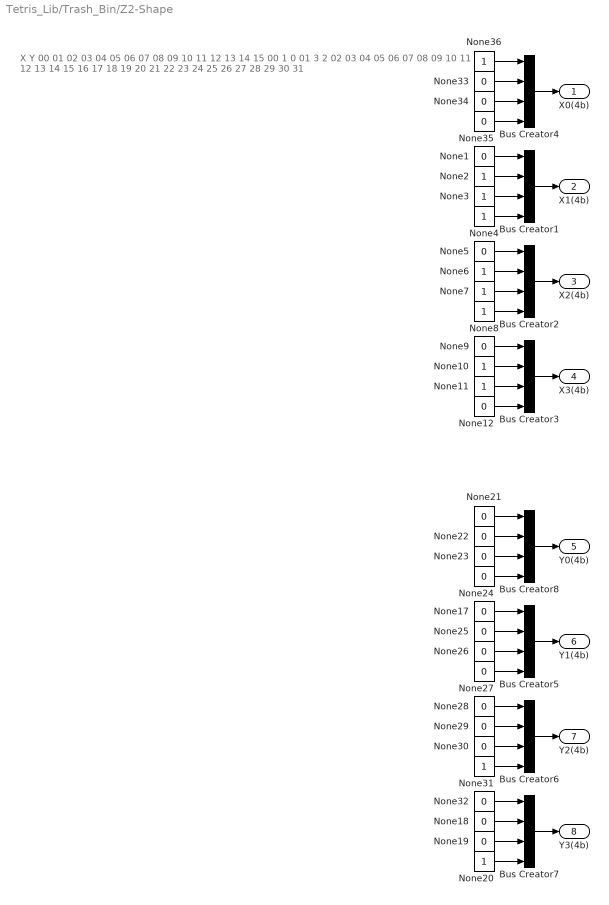
== system Tetris_Lib/Trash_Bin/Z2-Shape ==
  note: X
      |
      | Y
      |
      | 00
      | 01
      | 02
      | 03
      | 04
      | 05
      | 06
      | 07
      | 08
      | 09
      | 10
      | 11
      | 12
      | 13
      | 14
      | 15
      |
      | 00
      |
      | 1
      | 0
      |
      | 01
      |
      | 3
      | 2
      |
      | 02
      |
      | 03
      |
      | 04
      |
      | 05
      |
      | 06
      |
      | 07
      |
      | 08
      |
      | 09
      |
      | 10
      |
      | 11
      |
      | 12
      |
      | 13
      |
      | 14
      |
      | 15
      |
      | 16
      |
      | 17
      |
      | 18
      |
      | 19
      |
      | 20
      |
      | 21
      |
      | 22
      |
      | 23
      |
      | 24
      |
      | 25
      |
      | 26
      |
      | 27
      |
      | 28
      |
      | 29
      |
      | 30
      |
      | 31
  Bus Creator{1..8} (8 alike) : BusCreator  Inputs=4
  None{1,5,9,12,17..19,21..30,32..35} (21 alike) : Constant  Value=0  OutDataTypeStr=boolean
  None{2..4,6..8,10..11,20,31,36} (11 alike) : Constant  OutDataTypeStr=boolean
  X0(4b) : Outport
  X1(4b) : Outport  Port=2
  X2(4b) : Outport  Port=3
  X3(4b) : Outport  Port=4
  Y0(4b) : Outport  Port=5
  Y1(4b) : Outport  Port=6
  Y2(4b) : Outport  Port=7
  Y3(4b) : Outport  Port=8
  wires:
  None24/1 -> Bus Creator8/4
  None23/1 -> Bus Creator8/3
  None22/1 -> Bus Creator8/2
  None21/1 -> Bus Creator8/1
  Bus Creator8/1 -> Y0(4b)/1
  None20/1 -> Bus Creator7/4
  None19/1 -> Bus Creator7/3
  None18/1 -> Bus Creator7/2
  None32/1 -> Bus Creator7/1
  Bus Creator7/1 -> Y3(4b)/1
  None31/1 -> Bus Creator6/4
  None30/1 -> Bus Creator6/3
  None29/1 -> Bus Creator6/2
  None28/1 -> Bus Creator6/1
  Bus Creator6/1 -> Y2(4b)/1
  None27/1 -> Bus Creator5/4
  None26/1 -> Bus Creator5/3
  None25/1 -> Bus Creator5/2
  None17/1 -> Bus Creator5/1
  Bus Creator5/1 -> Y1(4b)/1
  None35/1 -> Bus Creator4/4
  None34/1 -> Bus Creator4/3
  None33/1 -> Bus Creator4/2
  None36/1 -> Bus Creator4/1
  Bus Creator4/1 -> X0(4b)/1
  None12/1 -> Bus Creator3/4
  None11/1 -> Bus Creator3/3
  None10/1 -> Bus Creator3/2
  None9/1 -> Bus Creator3/1
  Bus Creator3/1 -> X3(4b)/1
  None8/1 -> Bus Creator2/4
  None7/1 -> Bus Creator2/3
  None6/1 -> Bus Creator2/2
  None5/1 -> Bus Creator2/1
  Bus Creator2/1 -> X2(4b)/1
  None4/1 -> Bus Creator1/4
  None3/1 -> Bus Creator1/3
  None2/1 -> Bus Creator1/2
  None1/1 -> Bus Creator1/1
  Bus Creator1/1 -> X1(4b)/1

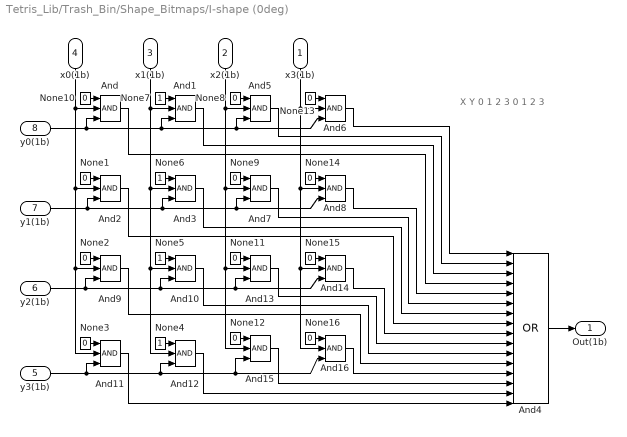
== system Tetris_Lib/Trash_Bin/Shape_Bitmaps/I-shape (0deg) ==
  note: X
      |
      | Y
      |
      | 0
      | 1
      | 2
      | 3
      |
      | 0
      |
      | 1
      |
      | 2
      |
      | 3
  x3(1b) : Inport
  x2(1b) : Inport  Port=2
  x1(1b) : Inport  Port=3
  x0(1b) : Inport  Port=4
  y3(1b) : Inport  Port=5
  y2(1b) : Inport  Port=6
  y1(1b) : Inport  Port=7
  y0(1b) : Inport  Port=8
  And{,1..3,5..16} (16 alike) : Logic  Inputs=3  IconShape=distinctive  AllPortsSameDT=off  OutDataTypeStr=boolean
  And4 : Logic  Operator=OR  Inputs=16  IconShape=distinctive  AllPortsSameDT=off  OutDataTypeStr=boolean
  None{1..3,8..16} (12 alike) : Constant  Value=0  OutDataTypeStr=boolean
  None{4..7} (4 alike) : Constant  OutDataTypeStr=boolean
  Out(1b) : Outport
  wires:
  y0(1b)/1 -> And/3, And1/3, And6/3, And5/3
  y1(1b)/1 -> And2/3, And3/3, And8/3, And7/3
  x0(1b)/1 -> And/2, And2/2, And11/2, And9/2
  x1(1b)/1 -> And1/2, And3/2, And12/2, And10/2
  And4/1 -> Out(1b)/1
  x2(1b)/1 -> And5/2, And7/2, And15/2, And13/2
  x3(1b)/1 -> And6/2, And8/2, And16/2, And14/2
  y2(1b)/1 -> And9/3, And10/3, And14/3, And13/3
  y3(1b)/1 -> And11/3, And12/3, And16/3, And15/3
  And6/1 -> And4/1
  And5/1 -> And4/2
  And1/1 -> And4/3
  And/1 -> And4/4
  And8/1 -> And4/5
  And7/1 -> And4/6
  And3/1 -> And4/7
  And2/1 -> And4/8
  And14/1 -> And4/9
  And13/1 -> And4/10
  And10/1 -> And4/11
  And9/1 -> And4/12
  And16/1 -> And4/13
  And15/1 -> And4/14
  And12/1 -> And4/15
  And11/1 -> And4/16
  None10/1 -> And/1
  None1/1 -> And2/1
  None2/1 -> And9/1
  None3/1 -> And11/1
  None4/1 -> And12/1
  None5/1 -> And10/1
  None6/1 -> And3/1
  None7/1 -> And1/1
  None8/1 -> And5/1
  None9/1 -> And7/1
  None11/1 -> And13/1
  None12/1 -> And15/1
  None13/1 -> And6/1
  None14/1 -> And8/1
  None15/1 -> And14/1
  None16/1 -> And16/1

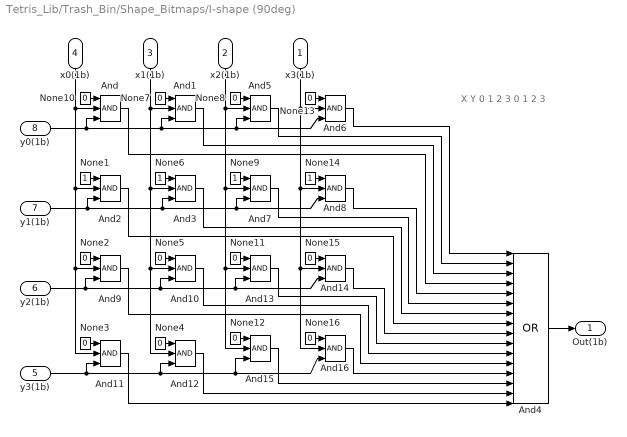
== system Tetris_Lib/Trash_Bin/Shape_Bitmaps/I-shape (90deg) ==
  note: X
      |
      | Y
      |
      | 0
      | 1
      | 2
      | 3
      |
      | 0
      |
      | 1
      |
      | 2
      |
      | 3
  x3(1b) : Inport
  x2(1b) : Inport  Port=2
  x1(1b) : Inport  Port=3
  x0(1b) : Inport  Port=4
  y3(1b) : Inport  Port=5
  y2(1b) : Inport  Port=6
  y1(1b) : Inport  Port=7
  y0(1b) : Inport  Port=8
  And{,1..3,5..16} (16 alike) : Logic  Inputs=3  IconShape=distinctive  AllPortsSameDT=off  OutDataTypeStr=boolean
  And4 : Logic  Operator=OR  Inputs=16  IconShape=distinctive  AllPortsSameDT=off  OutDataTypeStr=boolean
  None{1,6,9,14} (4 alike) : Constant  OutDataTypeStr=boolean
  None{2..5,7..8,10..13,15..16} (12 alike) : Constant  Value=0  OutDataTypeStr=boolean
  Out(1b) : Outport
  wires:
  y0(1b)/1 -> And/3, And1/3, And6/3, And5/3
  y1(1b)/1 -> And2/3, And3/3, And8/3, And7/3
  x0(1b)/1 -> And/2, And2/2, And11/2, And9/2
  x1(1b)/1 -> And1/2, And3/2, And12/2, And10/2
  And4/1 -> Out(1b)/1
  x2(1b)/1 -> And5/2, And7/2, And15/2, And13/2
  x3(1b)/1 -> And6/2, And8/2, And16/2, And14/2
  y2(1b)/1 -> And9/3, And10/3, And14/3, And13/3
  y3(1b)/1 -> And11/3, And12/3, And16/3, And15/3
  And6/1 -> And4/1
  And5/1 -> And4/2
  And1/1 -> And4/3
  And/1 -> And4/4
  And8/1 -> And4/5
  And7/1 -> And4/6
  And3/1 -> And4/7
  And2/1 -> And4/8
  And14/1 -> And4/9
  And13/1 -> And4/10
  And10/1 -> And4/11
  And9/1 -> And4/12
  And16/1 -> And4/13
  And15/1 -> And4/14
  And12/1 -> And4/15
  And11/1 -> And4/16
  None10/1 -> And/1
  None1/1 -> And2/1
  None2/1 -> And9/1
  None3/1 -> And11/1
  None4/1 -> And12/1
  None5/1 -> And10/1
  None6/1 -> And3/1
  None7/1 -> And1/1
  None8/1 -> And5/1
  None9/1 -> And7/1
  None11/1 -> And13/1
  None12/1 -> And15/1
  None13/1 -> And6/1
  None14/1 -> And8/1
  None15/1 -> And14/1
  None16/1 -> And16/1

== system Tetris_Lib/Trash_Bin/Shape_Bitmaps/L1-shape (0deg) ==
  note: X
      |
      | Y
      |
      | 0
      | 1
      | 2
      | 3
      |
      | 0
      |
      | 1
      |
      | 2
      |
      | 3
  x3(1b) : Inport
  x2(1b) : Inport  Port=2
  x1(1b) : Inport  Port=3
  x0(1b) : Inport  Port=4
  y3(1b) : Inport  Port=5
  y2(1b) : Inport  Port=6
  y1(1b) : Inport  Port=7
  y0(1b) : Inport  Port=8
  And{,1..3,5..16} (16 alike) : Logic  Inputs=3  IconShape=distinctive  AllPortsSameDT=off  OutDataTypeStr=boolean
  And4 : Logic  Operator=OR  Inputs=16  IconShape=distinctive  AllPortsSameDT=off  OutDataTypeStr=boolean
  None{1..2,5,10} (4 alike) : Constant  OutDataTypeStr=boolean
  None{3..4,6..9,11..16} (12 alike) : Constant  Value=0  OutDataTypeStr=boolean
  Out(1b) : Outport
  wires:
  y0(1b)/1 -> And/3, And1/3, And6/3, And5/3
  y1(1b)/1 -> And2/3, And3/3, And8/3, And7/3
  x0(1b)/1 -> And/2, And2/2, And11/2, And9/2
  x1(1b)/1 -> And1/2, And3/2, And12/2, And10/2
  And4/1 -> Out(1b)/1
  x2(1b)/1 -> And5/2, And7/2, And15/2, And13/2
  x3(1b)/1 -> And6/2, And8/2, And16/2, And14/2
  y2(1b)/1 -> And9/3, And10/3, And14/3, And13/3
  y3(1b)/1 -> And11/3, And12/3, And16/3, And15/3
  And6/1 -> And4/1
  And5/1 -> And4/2
  And1/1 -> And4/3
  And/1 -> And4/4
  And8/1 -> And4/5
  And7/1 -> And4/6
  And3/1 -> And4/7
  And2/1 -> And4/8
  And14/1 -> And4/9
  And13/1 -> And4/10
  And10/1 -> And4/11
  And9/1 -> And4/12
  And16/1 -> And4/13
  And15/1 -> And4/14
  And12/1 -> And4/15
  And11/1 -> And4/16
  None10/1 -> And/1
  None1/1 -> And2/1
  None2/1 -> And9/1
  None3/1 -> And11/1
  None4/1 -> And12/1
  None5/1 -> And10/1
  None6/1 -> And3/1
  None7/1 -> And1/1
  None8/1 -> And5/1
  None9/1 -> And7/1
  None11/1 -> And13/1
  None12/1 -> And15/1
  None13/1 -> And6/1
  None14/1 -> And8/1
  None15/1 -> And14/1
  None16/1 -> And16/1
